simulink model "StanleyRefMdl"  (R2021b)
settings: Solver=FixedStepAuto  StartTime=0.0  StopTime=inf  FixedStep=0.05  MaxStep=1e-2  MinStep=1e-3  RelTol=5e-3
libraries: drivingvehiclecontroller x2
settings Model: Creator=The MathWorks, Inc.  LastModifiedBy=Asus ROG
settings SolverCC: ZeroCrossAlgorithm=Adaptive  AlgebraicLoopSolver=TrustRegion  DecoupledContinuousIntegration=on  MinimalZcImpactIntegration=on
settings DataIOCC: SaveOutput=off  SignalLogging=off  DSMLogging=off  SaveTime=off  ReturnWorkspaceOutputs=off
settings DebuggingCC: PregeneratedLibrarySubsystemCodeDiagnostic=none  SFMachineParentedDataDiag=warning  ArithmeticOperatorsInVariantConditions=warning
settings SFSimCC: SimUseLocalCustomCode=off
settings RTWCC: RTWUseLocalCustomCode=off

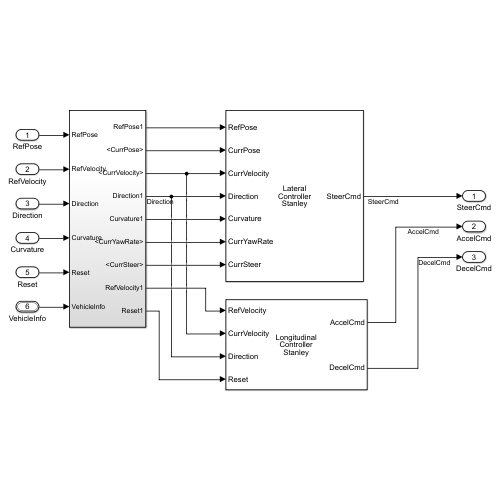
[thumbnail: Simulink's stored preview of the top-level diagram]
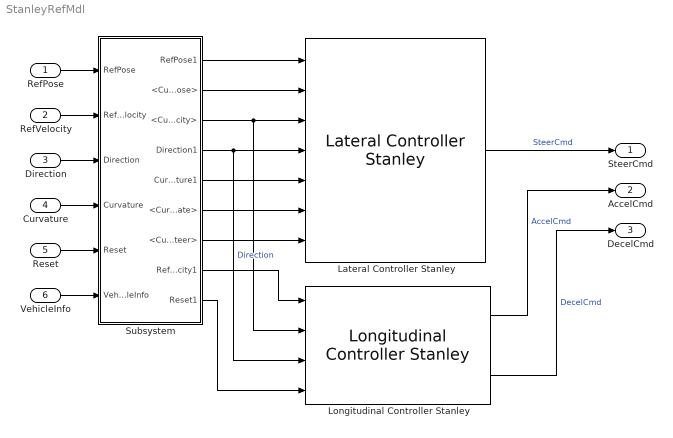
== system StanleyRefMdl ==
  RefPose : Inport  OutDataTypeStr=double  PortDimensions=[1 3]  SampleTime=[0.050000000000000003,0]
  RefVelocity : Inport  Port=2  OutDataTypeStr=double  PortDimensions=[1 1]  SampleTime=[0.050000000000000003,0]
  Direction : Inport  Port=3  OutDataTypeStr=double  PortDimensions=[1 1]  SampleTime=[0.050000000000000003,0]
  Curvature : Inport  Port=4  OutDataTypeStr=double  PortDimensions=[1 1]  SampleTime=[0.050000000000000003,0]
  Reset : Inport  Port=5  OutDataTypeStr=double  PortDimensions=[1 1]  SampleTime=[0.050000000000000003,0]
  VehicleInfo : Inport  Port=6  OutDataTypeStr=Bus: vehicleInfoBus
  Lateral Controller Stanley : drivingvehiclecontroller/Lateral Controller Stanley  ModelType=Dynamic bicycle model  PositionGainF=2  PositionGainR=2.5  YawRateGain=0.25  DelayGain=0.2  VehicleMass=1575  Lf=1.4  Lr=1.4  TireStiffness=19000  Wheelbase=2.8  MaxSteeringAngle=35
      settings: SourceProductBaseCode=DR
  Longitudinal Controller Stanley : drivingvehiclecontroller/Longitudinal Controller Stanley  Kp=2.5  Ki=1  SampleTime=0.05  MaxAcceleration=3  MaxDeceleration=6
      settings: SourceProductBaseCode=DR
  Subsystem : Subsystem
  SteerCmd : Outport  VectorParamsAs1DForOutWhenUnconnected=off
  AccelCmd : Outport  Port=2  VectorParamsAs1DForOutWhenUnconnected=off
  DecelCmd : Outport  Port=3  VectorParamsAs1DForOutWhenUnconnected=off
  wires:
  Lateral Controller Stanley/1 -> SteerCmd/1  "SteerCmd"
  Longitudinal Controller Stanley/1 -> AccelCmd/1  "AccelCmd"
  Longitudinal Controller Stanley/2 -> DecelCmd/1  "DecelCmd"
  RefPose/1 -> Subsystem/1(RefPose)
  RefVelocity/1 -> Subsystem/2(RefVelocity)
  Direction/1 -> Subsystem/3(Direction)
  Curvature/1 -> Subsystem/4(Curvature)
  Reset/1 -> Subsystem/5(Reset)
  VehicleInfo/1 -> Subsystem/6(VehicleInfo)
  Subsystem/1(RefPose1) -> Lateral Controller Stanley/1
  Subsystem/3(<CurrVelocity>) -> Lateral Controller Stanley/3, Longitudinal Controller Stanley/2
  Subsystem/4(Direction1) -> Longitudinal Controller Stanley/3, Lateral Controller Stanley/4  "Direction"
  Subsystem/8(RefVelocity1) -> Longitudinal Controller Stanley/1
  Subsystem/9(Reset1) -> Longitudinal Controller Stanley/4
  Subsystem/6(<CurrYawRate>) -> Lateral Controller Stanley/6
  Subsystem/7(<CurrSteer>) -> Lateral Controller Stanley/7
  Subsystem/2(<CurrPose>) -> Lateral Controller Stanley/2
  Subsystem/5(Curvature1) -> Lateral Controller Stanley/5

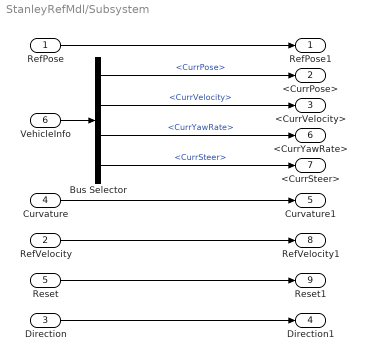
== system StanleyRefMdl/Subsystem ==
  RefPose : Inport
  RefVelocity : Inport  Port=2
  Direction : Inport  Port=3
  Curvature : Inport  Port=4
  Reset : Inport  Port=5
  VehicleInfo : Inport  Port=6
  Bus Selector : BusSelector  OutputSignals=CurrPose,CurrVelocity,CurrYawRate,CurrSteer
  RefPose1 : Outport  VectorParamsAs1DForOutWhenUnconnected=off
  <CurrPose> : Outport  Port=2  VectorParamsAs1DForOutWhenUnconnected=off
  <CurrVelocity> : Outport  Port=3  VectorParamsAs1DForOutWhenUnconnected=off
  Direction1 : Outport  Port=4  VectorParamsAs1DForOutWhenUnconnected=off
  Curvature1 : Outport  Port=5  VectorParamsAs1DForOutWhenUnconnected=off
  <CurrYawRate> : Outport  Port=6  VectorParamsAs1DForOutWhenUnconnected=off
  <CurrSteer> : Outport  Port=7  VectorParamsAs1DForOutWhenUnconnected=off
  RefVelocity1 : Outport  Port=8  VectorParamsAs1DForOutWhenUnconnected=off
  Reset1 : Outport  Port=9  VectorParamsAs1DForOutWhenUnconnected=off
  wires:
  Bus Selector/4 -> <CurrSteer>/1  "<CurrSteer>"
  Curvature/1 -> Curvature1/1
  Bus Selector/3 -> <CurrYawRate>/1  "<CurrYawRate>"
  Reset/1 -> Reset1/1
  RefPose/1 -> RefPose1/1
  Bus Selector/1 -> <CurrPose>/1  "<CurrPose>"
  Bus Selector/2 -> <CurrVelocity>/1  "<CurrVelocity>"
  RefVelocity/1 -> RefVelocity1/1
  VehicleInfo/1 -> Bus Selector/1
  Direction/1 -> Direction1/1
